simulink model "Landing"  (R2016a)
settings: Solver=VariableStepAuto  StartTime=0.0  StopTime=420  FixedStep=0.01  RelTol=1e-3
libraries: simulink x3
settings Model: Creator=jason  LastModifiedBy=jason
settings SolverCC: ZeroCrossAlgorithm=Adaptive
settings GRTTargetCC: GeneratePreprocessorConditionals=Use local settings

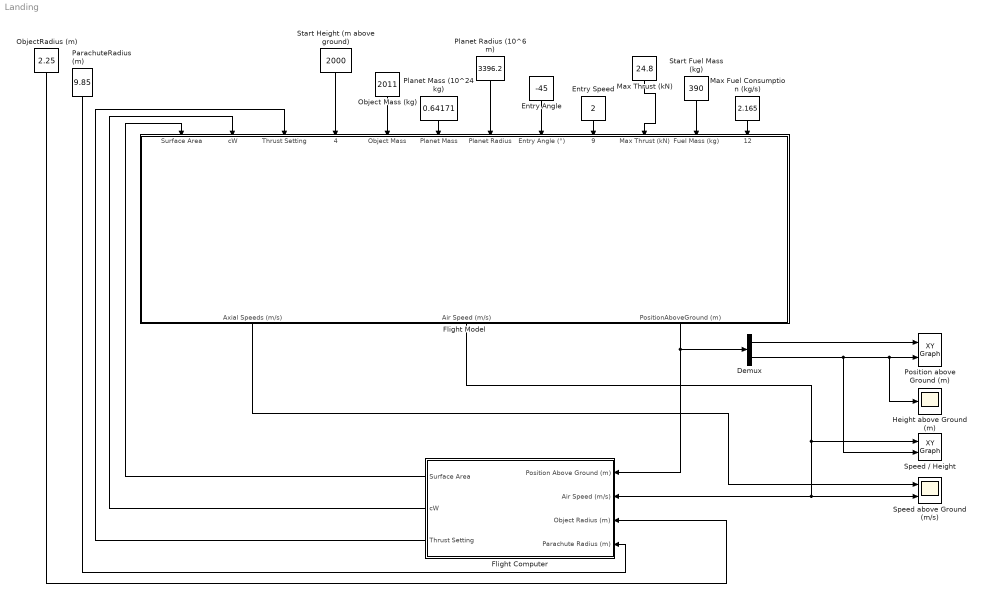
== system Landing ==
  Demux : Demux  Outputs=2
  Entry Angle : Constant  Value=-45
  Entry Speed : Constant  Value=2
  Flight Computer : Subsystem
  Flight Model : Subsystem
  Height above Ground (m) : Scope
  Max Fuel Consumption (kg/s) : Constant  Value=2.165
  Max Thrust (kN) : Constant  Value=24.8
  Object Mass (kg) : Constant  Value=2011
  ObjectRadius (m) : Constant  Value=2.25
  ParachuteRadius (m) : Constant  Value=9.85
  Planet Mass (10^24 kg) : Constant  Value=0.64171
  Planet Radius (10^6 m) : Constant  Value=3396.2
  Position above Ground (m) : simulink/Sinks/XY Graph  xmin=0  xmax=500000  ymin=0  ymax=130000  st=-1
  Speed / Height : simulink/Sinks/XY Graph  xmin=0  xmax=5800  ymin=0  ymax=130000  st=-1
  Speed above Ground (m/s) : Scope  NumInputPorts=2
  Start Fuel Mass (kg) : Constant  Value=390
  Start Height (m above ground) : Constant  Value=2000
  wires:
  Planet Mass (10^24 kg)/1 -> Flight Model/6(Planet Mass)
  Object Mass (kg)/1 -> Flight Model/5(Object Mass)
  Planet Radius (10^6 m)/1 -> Flight Model/7(Planet Radius)
  Start Height (m above ground)/1 -> Flight Model/4(Start Height (m above ground))
  Flight Model/3(PositionAboveGround (m)) -> Demux/1, Flight Computer/1(Position Above Ground (m))
  Demux/1 -> Position above Ground (m)/1
  Demux/2 -> Height above Ground (m)/1, Position above Ground (m)/2, Speed / Height/2
  Entry Angle/1 -> Flight Model/8(Entry Angle (°))
  Entry Speed/1 -> Flight Model/9(Entry Speed (m/s))
  Flight Model/2(Air Speed (m/s)) -> Flight Computer/2(Air Speed (m/s)), Speed above Ground (m/s)/2, Speed / Height/1
  Flight Computer/2(cW) -> Flight Model/2(cW)
  ParachuteRadius (m)/1 -> Flight Computer/4(Parachute Radius (m))
  ObjectRadius (m)/1 -> Flight Computer/3(Object Radius (m))
  Flight Model/1(Axial Speeds (m/s)) -> Speed above Ground (m/s)/1
  Max Thrust (kN)/1 -> Flight Model/10(Max Thrust (kN))
  Flight Computer/3(Thrust Setting) -> Flight Model/3(Thrust Setting)
  Start Fuel Mass (kg)/1 -> Flight Model/11(Fuel Mass (kg))
  Max Fuel Consumption (kg/s)/1 -> Flight Model/12(Max Fuel Consumption (kg/s))
  Flight Computer/1(Surface Area) -> Flight Model/1(Surface Area)

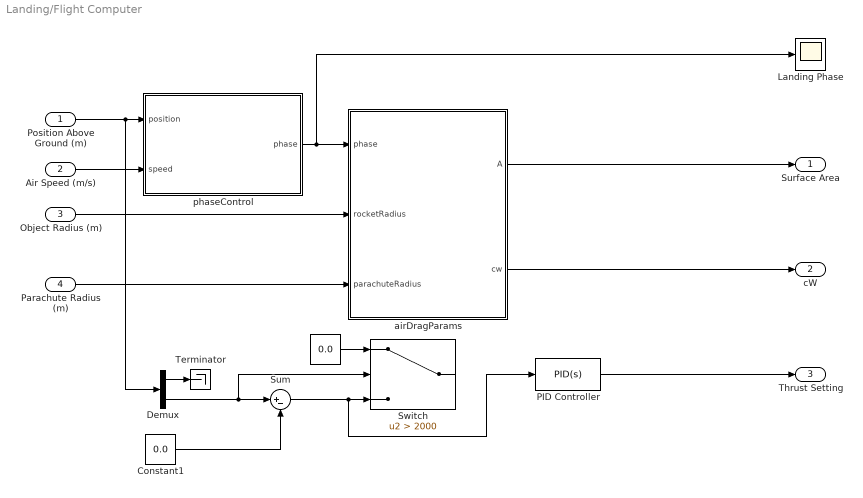
== system Landing/Flight Computer ==
  Position Above Ground (m) : Inport
  Air Speed (m/s) : Inport  Port=2
  Object Radius (m) : Inport  Port=3
  Parachute Radius (m) : Inport  Port=4
  " " : Constant  Value=0.0
  Constant1 : Constant  Value=0.0
  Demux : Demux  Outputs=2
  Landing Phase : Scope
  PID Controller : simulink/Continuous/PID Controller  Controller=PID  TimeDomain=Continuous-time  SampleTime=-1  IntegratorMethod=Forward Euler  FilterMethod=Forward Euler  Form=Parallel  UseFilter=on  ControllerParametersSource=internal  P=-0.0655908001368762  I=-0.00191326031997097  D=-0.499611888952789  N=571.413988020802  InitialConditionSource=internal  InitialConditionForIntegrator=0  InitialConditionForFilter=0  ExternalReset=none  LimitOutput=on  UpperSaturationLimit=1.0  LowerSaturationLimit=0.0  LinearizeAsGain=on  AntiWindupMode=back-calculation  Kb=5  TrackingMode=off  Kt=1  PParamMin=[]  PParamMax=[]  IParamMin=[]  IParamMax=[]  DParamMin=[]  DParamMax=[]  NParamMin=[]  NParamMax=[]  KbParamMin=[]  KbParamMax=[]  KtParamMin=[]  KtParamMax=[]  POutMin=[]  POutMax=[]  IOutMin=[]  IOutMax=[]  DOutMin=[]  DOutMax=[]  NOutMin=[]  NOutMax=[]  KbOutMin=[]  KbOutMax=[]  KtOutMin=[]  KtOutMax=[]  IntegratorOutMin=[]  IntegratorOutMax=[]  FilterOutMin=[]  FilterOutMax=[]  SumOutMin=[]  SumOutMax=[]  SumI1OutMin=[]  SumI1OutMax=[]  SumI2OutMin=[]  SumI2OutMax=[]  SumI3OutMin=[]  SumI3OutMax=[]  SumDOutMin=[]  SumDOutMax=[]  SaturationOutMin=[]  SaturationOutMax=[]  IntegratorContinuousStateAttributes=''  IntegratorStateMustResolveToSignalObject=off  IntegratorRTWStateStorageClass=Auto  FilterContinuousStateAttributes=''  FilterStateMustResolveToSignalObject=off  FilterRTWStateStorageClass=Auto  DifferentiatorICPrevScaledInput=0  DifferentiatorOutMin=[]  DifferentiatorOutMax=[]
  Sum : Sum  Inputs=|+-
  Switch : Switch  Criteria=u2 > Threshold  Threshold=2000
  Terminator : Terminator
  airDragParams : MATLAB Function  TreatAsAtomicUnit=on
  phaseControl : MATLAB Function  TreatAsAtomicUnit=on
  Surface Area : Outport
  cW : Outport  Port=2
  Thrust Setting : Outport  Port=3
  wires:
  Position Above Ground (m)/1 -> phaseControl/1(position), Demux/1
  airDragParams/2(cw) -> cW/1
  airDragParams/1(A) -> Surface Area/1
  Object Radius (m)/1 -> airDragParams/2(rocketRadius)
  Parachute Radius (m)/1 -> airDragParams/3(parachuteRadius)
  Air Speed (m/s)/1 -> phaseControl/2(speed)
  Constant1/1 -> Sum/2
  Demux/2 -> Switch/2, Sum/1
  Sum/1 -> PID Controller/1, Switch/3
  phaseControl/1(phase) -> Landing Phase/1, airDragParams/1(phase)
  " "/1 -> Switch/1
  Demux/1 -> Terminator/1
  PID Controller/1 -> Thrust Setting/1

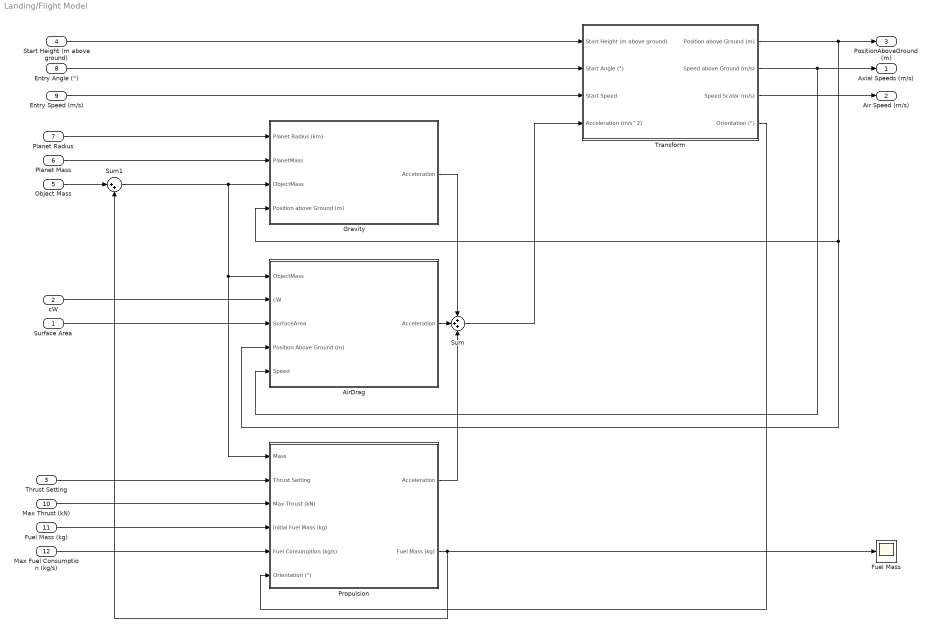
== system Landing/Flight Model ==
  Surface Area : Inport
  cW : Inport  Port=2
  Thrust Setting : Inport  Port=3
  Start Height (m above ground) : Inport  Port=4
  Object Mass : Inport  Port=5
  Planet Mass : Inport  Port=6
  Planet Radius : Inport  Port=7
  Entry Angle (°) : Inport  Port=8
  Entry Speed (m/s) : Inport  Port=9
  Max Thrust (kN) : Inport  Port=10
  Fuel Mass (kg) : Inport  Port=11
  Max Fuel Consumption (kg/s) : Inport  Port=12
  AirDrag : Subsystem
  Fuel Mass : Scope
  Gravity : Subsystem
  Propulsion : Subsystem
  Sum : Sum  Inputs=+++  OutDataTypeStr=Inherit: Same as first input
  Sum1 : Sum  Inputs=|++
  Transform : Subsystem
  Axial Speeds (m/s) : Outport
  Air Speed (m/s) : Outport  Port=2
  PositionAboveGround (m) : Outport  Port=3
  wires:
  Planet Mass/1 -> Gravity/2(PlanetMass)
  Object Mass/1 -> Sum1/1
  Planet Radius/1 -> Gravity/1(Planet Radius (km))
  cW/1 -> AirDrag/2(cW)
  Surface Area/1 -> AirDrag/3(SurfaceArea)
  Max Thrust (kN)/1 -> Propulsion/3(Max Thrust (kN))
  Thrust Setting/1 -> Propulsion/2(Thrust Setting)
  AirDrag/1("Acceleration ") -> Sum/2
  Gravity/1(Acceleration) -> Sum/1
  Start Height (m above ground)/1 -> Transform/1(Start Height (m above ground))
  Entry Speed (m/s)/1 -> Transform/3(Start Speed)
  Entry Angle (°)/1 -> Transform/2(Start Angle (°))
  Sum/1 -> Transform/4(Acceleration (m/s^2))
  Transform/1(Position above Ground (m)) -> Gravity/4(Position above Ground (m)), AirDrag/4(Position Above Ground (m)), PositionAboveGround (m)/1
  Transform/2(Speed above Ground (m/s)) -> AirDrag/5(Speed), Axial Speeds (m/s)/1
  Transform/3(Speed Scalar (m/s)) -> Air Speed (m/s)/1
  Transform/4(Orientation (°)) -> Propulsion/6(Orientation (°))
  Propulsion/1(Acceleration) -> Sum/3
  Fuel Mass (kg)/1 -> Propulsion/4(Initial Fuel Mass (kg))
  Max Fuel Consumption (kg/s)/1 -> Propulsion/5(Fuel Consumption (kg/s))
  Sum1/1 -> Gravity/3(ObjectMass), Propulsion/1(Mass), AirDrag/1(ObjectMass)
  Propulsion/2(Fuel Mass (kg)) -> Sum1/2, Fuel Mass/1

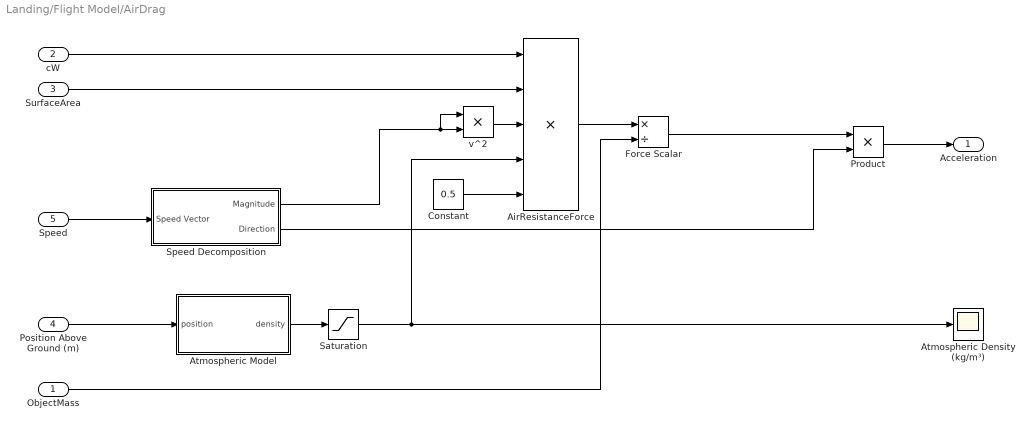
== system Landing/Flight Model/AirDrag ==
  ObjectMass : Inport
  cW : Inport  Port=2
  SurfaceArea : Inport  Port=3
  Position Above Ground (m) : Inport  Port=4
  Speed : Inport  Port=5
  AirResistanceForce : Product  Inputs=5
  Atmospheric Density (kg/m³) : Scope
  Atmospheric Model : MATLAB Function  TreatAsAtomicUnit=on
  Constant : Constant  Value=0.5
  Force Scalar : Product  Inputs=*/
  Product : Product
  Saturation : Saturate  UpperLimit=0.02  LowerLimit=0
  Speed Decomposition : Subsystem
  v^2 : Product
  "Acceleration " : Outport
  wires:
  Speed/1 -> Speed Decomposition/1(Speed Vector)
  SurfaceArea/1 -> AirResistanceForce/2
  v^2/1 -> AirResistanceForce/3
  Constant/1 -> AirResistanceForce/5
  Position Above Ground (m)/1 -> Atmospheric Model/1(position)
  Atmospheric Model/1(density) -> Saturation/1
  Speed Decomposition/1(Magnitude) -> v^2/1, v^2/2
  AirResistanceForce/1 -> Force Scalar/1
  ObjectMass/1 -> Force Scalar/2
  Speed Decomposition/2(Direction) -> Product/2
  Product/1 -> "Acceleration "/1
  cW/1 -> AirResistanceForce/1
  Force Scalar/1 -> Product/1
  Saturation/1 -> AirResistanceForce/4, Atmospheric Density (kg/m³)/1

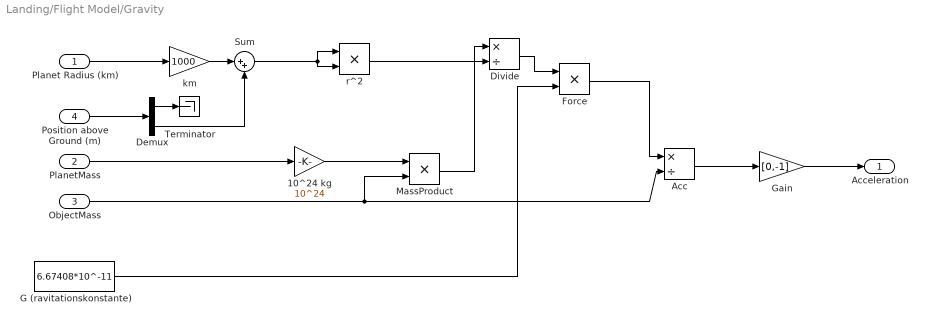
== system Landing/Flight Model/Gravity ==
  Planet Radius (km) : Inport
  PlanetMass : Inport  Port=2
  ObjectMass : Inport  Port=3
  Position above Ground (m) : Inport  Port=4
  10^24 kg : Gain  Gain=10^24
  Acc : Product  Inputs=*/
  Demux : Demux  Outputs=2
  Divide : Product  Inputs=*/
  Force : Product
  G (ravitationskonstante) : Constant  Value=6.67408*10^-11
  Gain : Gain  Gain=[0,-1]
  MassProduct : Product
  Sum : Sum  Inputs=|++
  Terminator : Terminator
  km : Gain  Gain=1000
  r^2 : Product
  Acceleration : Outport
  wires:
  MassProduct/1 -> Divide/1
  r^2/1 -> Divide/2
  Divide/1 -> Force/1
  G (ravitationskonstante)/1 -> Force/2
  Force/1 -> Acc/1
  ObjectMass/1 -> MassProduct/2, Acc/2
  Acc/1 -> Gain/1
  Gain/1 -> Acceleration/1
  PlanetMass/1 -> 10^24 kg/1
  10^24 kg/1 -> MassProduct/1
  Sum/1 -> r^2/1, r^2/2
  Position above Ground (m)/1 -> Demux/1
  Demux/2 -> Sum/2
  km/1 -> Sum/1
  Planet Radius (km)/1 -> km/1
  Demux/1 -> Terminator/1

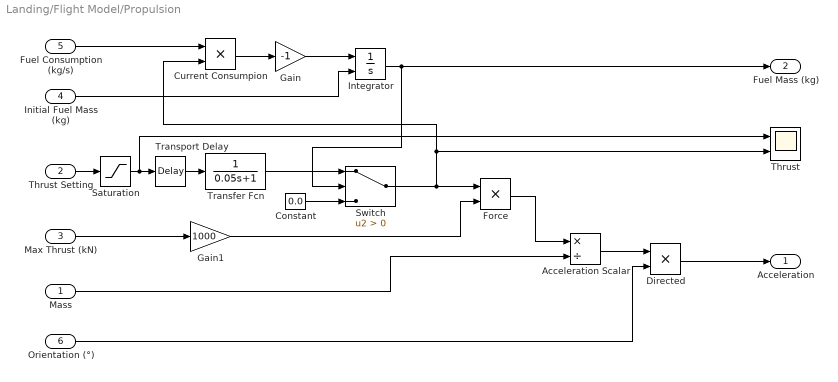
== system Landing/Flight Model/Propulsion ==
  Mass : Inport
  Thrust Setting : Inport  Port=2
  Max Thrust (kN) : Inport  Port=3
  Initial Fuel Mass (kg) : Inport  Port=4
  Fuel Consumption (kg/s) : Inport  Port=5
  Orientation (°) : Inport  Port=6
  Acceleration Scalar : Product  Inputs=*/
  Constant : Constant  Value=0.0
  Current Consumpion : Product
  Directed : Product
  Force : Product
  Gain : Gain  Gain=-1
  Gain1 : Gain  Gain=1000
  Integrator : Integrator  InitialConditionSource=external
  Saturation : Saturate  UpperLimit=1  LowerLimit=0
  Switch : Switch  Criteria=u2 > Threshold
  Thrust : Scope  NumInputPorts=2
  Transfer Fcn : TransferFcn  Denominator=[0.05 1]
  Transport Delay : TransportDelay  DelayTime=0.1
  Acceleration : Outport
  Fuel Mass (kg) : Outport  Port=2
  wires:
  Mass/1 -> Acceleration Scalar/2
  Force/1 -> Acceleration Scalar/1
  Directed/1 -> Acceleration/1
  Max Thrust (kN)/1 -> Gain1/1
  Gain1/1 -> Force/2
  Acceleration Scalar/1 -> Directed/1
  Orientation (°)/1 -> Directed/2
  Transfer Fcn/1 -> Switch/1
  Transport Delay/1 -> Transfer Fcn/1
  Initial Fuel Mass (kg)/1 -> Integrator/2
  Fuel Consumption (kg/s)/1 -> Current Consumpion/1
  Current Consumpion/1 -> Gain/1
  Gain/1 -> Integrator/1
  Integrator/1 -> Fuel Mass (kg)/1, Switch/2
  Switch/1 -> Current Consumpion/2, Thrust/2, Force/1
  Constant/1 -> Switch/3
  Saturation/1 -> Thrust/1, Transport Delay/1
  Thrust Setting/1 -> Saturation/1

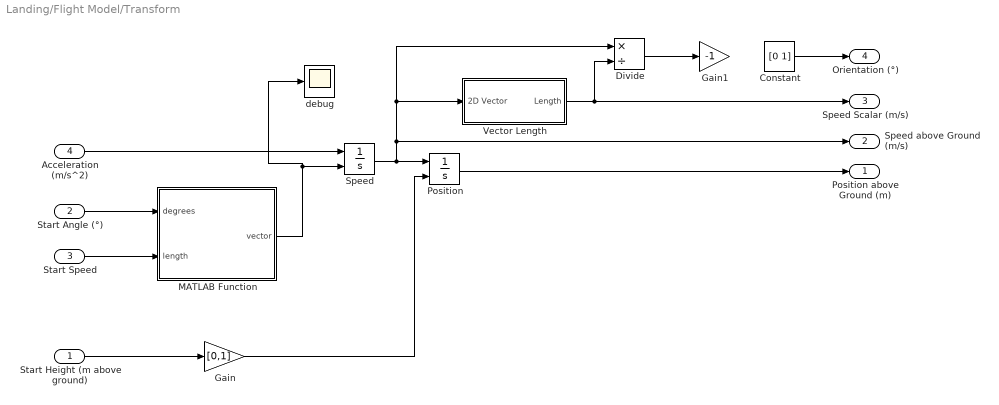
== system Landing/Flight Model/Transform ==
  Start Height (m above ground) : Inport
  Start Angle (°) : Inport  Port=2
  Start Speed : Inport  Port=3
  Acceleration (m/s^2) : Inport  Port=4
  Constant : Constant  Value=[0 1]
  Divide : Product  Inputs=*/
  Gain : Gain  Gain=[0,1]
  Gain1 : Gain  Gain=-1
  MATLAB Function : MATLAB Function  TreatAsAtomicUnit=on
  Position : Integrator  InitialConditionSource=external
  Speed : Integrator  InitialConditionSource=external  InitialCondition=[20, 0]
  Vector Length : Subsystem
  debug : Scope
  Position above Ground (m) : Outport
  Speed above Ground (m/s) : Outport  Port=2
  Speed Scalar (m/s) : Outport  Port=3
  Orientation (°) : Outport  Port=4
  wires:
  Start Height (m above ground)/1 -> Gain/1
  Gain/1 -> Position/2
  Start Angle (°)/1 -> MATLAB Function/1(degrees)
  Start Speed/1 -> MATLAB Function/2(length)
  MATLAB Function/1(vector) -> debug/1, Speed/2
  Acceleration (m/s^2)/1 -> Speed/1
  Speed/1 -> Position/1, Vector Length/1(2D Vector), Divide/1, Speed above Ground (m/s)/1
  Position/1 -> Position above Ground (m)/1
  Vector Length/1(Length) -> Divide/2, Speed Scalar (m/s)/1
  Divide/1 -> Gain1/1
  Constant/1 -> Orientation (°)/1

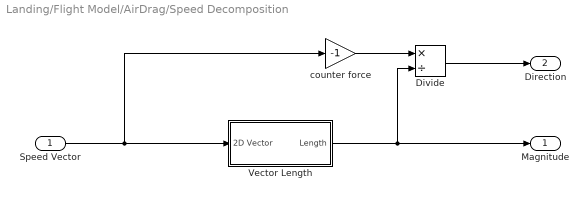
== system Landing/Flight Model/AirDrag/Speed Decomposition ==
  Speed Vector : Inport
  Divide : Product  Inputs=*/
  Vector Length : Subsystem
  counter force : Gain  Gain=-1
  Magnitude : Outport
  Direction : Outport  Port=2
  wires:
  Speed Vector/1 -> Vector Length/1(2D Vector), counter force/1
  Divide/1 -> Direction/1
  counter force/1 -> Divide/1
  Vector Length/1(Length) -> Divide/2, Magnitude/1

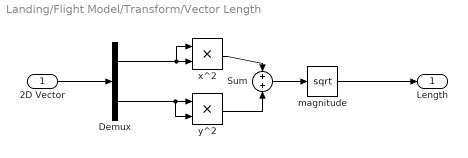
== system Landing/Flight Model/Transform/Vector Length ==
  2D Vector : Inport
  Demux : Demux  Outputs=2
  Sum : Sum  Inputs=+|+
  magnitude : Sqrt  SaturateOnIntegerOverflow=on
  x^2 : Product
  y^2 : Product
  Length : Outport
  wires:
  2D Vector/1 -> Demux/1
  magnitude/1 -> Length/1
  Demux/2 -> y^2/2, y^2/1
  Demux/1 -> x^2/1, x^2/2
  x^2/1 -> Sum/1
  y^2/1 -> Sum/2
  Sum/1 -> magnitude/1

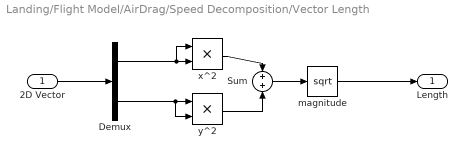
== system Landing/Flight Model/AirDrag/Speed Decomposition/Vector Length ==
  2D Vector : Inport
  Demux : Demux  Outputs=2
  Sum : Sum  Inputs=+|+
  magnitude : Sqrt  SaturateOnIntegerOverflow=on
  x^2 : Product
  y^2 : Product
  Length : Outport
  wires:
  2D Vector/1 -> Demux/1
  magnitude/1 -> Length/1
  Demux/2 -> y^2/2, y^2/1
  Demux/1 -> x^2/1, x^2/2
  x^2/1 -> Sum/1
  y^2/1 -> Sum/2
  Sum/1 -> magnitude/1

== matlab function Landing/Flight Model/AirDrag/Atmospheric Model ==
  data: position input; density output
function density   = Density( position )
% result is gas density in kg * m^3 
   height = position(2);
   p = 0.699 * exp(-0.00009 * height);
   
   if height > 7000
       T = -23.4 - 0.00222 * height;       
   else
       T = -31 - 0.000998 * height;       
   end
   
   %density = p / (0.1921 * (T + 273.1));
   density = p / (0.147 * (T + 273.1));
end

== matlab function Landing/Flight Computer/airDragParams ==
  data: phase input; A output; rocketRadius input; cw output; parachuteRadius input
function [A, cw] = airDragParameters(phase, rocketRadius, parachuteRadius)

    if phase == 1
        A = area(parachuteRadius);
        cw = 1.33;
    else        
        A = area(rocketRadius);
        cw = 0.34;
    end
end

function A = area( radius )
    A = 3.14159 * radius * radius;
end

== matlab function Landing/Flight Computer/phaseControl ==
  data: position input; phase output; speed input
function phase = phaseControl(position, speed)
    persistent stage;
    if isempty(stage)
        stage = 0;
    end
    
    switch stage
        case 0
            phase = hypersonicEntry(position, speed);
            stage = phase;
        case 1
            phase = parachute(position);
            stage = phase;
        case 2
            phase = poweredDescent(position, speed);
            stage = phase;
        otherwise
            error('Flight Controller is in unknown phase.');
    end
end

function phase = hypersonicEntry(position, speed)
    if position(2) <= 15000 || speed <= 1000
        phase = 1;
    else
        phase = 0;
    end
end

function phase = parachute(position)
    if position(2) <= 2000
        phase = 2;
    else
        phase = 1;
    end
end

function phase = poweredDescent(position, speed)
    if position(2) <= 0.05
        if speed <= 1.5
            error('Soft Touchdown. Speed: %.3f', speed);
        else
            error('Hard Drop/Crash. Speed: %.3f', speed);
        end
        phase = 2;
    else
        phase = 2;
    end
end

== matlab function Landing/Flight Model/Transform/MATLAB Function ==
  data: degrees input; vector output; length input
function vector = vectorize(degrees, length)
    degreesToRad = 3.14159 / 180;
    
    radAngle = degreesToRad * degrees;
    
    x = cos(radAngle);
    y = sin(radAngle);
    vector = [x, y] * length;
